simulink library "DsmCheatRead"  (R2022b)
settings: Solver=VariableStepAuto  StartTime=0.0  StopTime=10.0  RelTol=1e-3
values from neighbouring files (symbols this model uses):
  dsmIdentifier = dsmName    [DsmCheatReadConfig.m]
libraries: HandyTextFile x1
settings Model: Creator=kl13806  LastModifiedBy=kl13806
settings SolverCC: AlgebraicLoopSolver=TrustRegion
settings DebuggingCC: UnconnectedInputMsg=warning  UnconnectedOutputMsg=warning  UnconnectedLineMsg=warning  SFMachineParentedDataDiag=warning
settings ModelReferenceCC: EnableRefExpFcnMdlSchedulingChecks=on

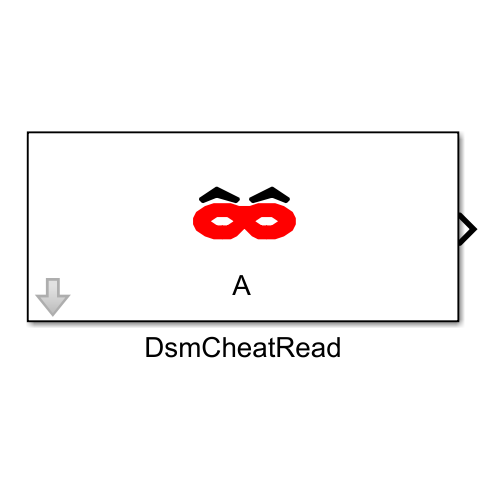
[thumbnail: Simulink's stored preview of the top-level diagram]
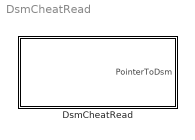
== system DsmCheatRead ==
  DsmCheatRead : Subsystem  mask{DataStoreName=A, Config=[], TriggerInit=0}
      mask prompts: DataStoreName "Simulink:blkprm_prompts:DstoreMemDstoreName"; Config "DsmCheatReadConfig"; TriggerInit "Used to trigger initialization"
      mask init:
      | blkh=gcbh;
      | Config=BTConfig.Assert(blkh,Config);
      | 
      | Config.Validate();
      | 
      | Config.DoMaskInit(blkh);
      settings: MoveFcn=DsmCheatReadConfig.CbTriggerInit(gcbh);
      mask TypeOptions DataStoreName:
      | DsmAccess/Data Store
      | Read/DataStoreName
      mask DialogControl DataStoreName Prompt: Data store name:
      mask DialogControl InfoText Prompt: Registered DSM:
      mask DialogControl RegisteredDsmName Prompt: A
      mask DialogControl ButtonRegister Prompt: Re-register DSM
      mask DialogControl ButtonRegister Callback: DsmCheatReadConfig.CbButtonRegister(gcbh);
      mask Display:
      | % retrieve icon definition
      | [path,w,h] = DsmCheatReadConfig.Icon();
      | 
      | % retrieve the block's pixel size
      | pos = get(gcbh,'position');
      | bw = pos(3) - pos(1);
      | bh = pos(4) - pos(2);
      | 
      | % draw centered icon
      | xAdj = bw/2 - w/2;
      | yAdj = bh/2 - h/2 + 5;
      | for i=1:length(path)
      |    if (path(i).rgb(1) >= 0)
      |       patch(path(i).x+xAdj, path(i).y+yAdj, path(i).rgb);
      |    end
      |    if (path(i).stroke(1) >= 0)
      |       plot(path(i).x+xAdj, path(i).y+yAdj);
      |    end
      | end
      | 
      | % show the name or an X
      | if (true)
      |     text(bw*0.5, bh*0.2, DataStoreName, 'horizontalAlignment','center');
      | 	patch(0,0,[1 1 1]);
      | 	patch(bw,bh,[1 1 1]);
      | else
      | 	tx=bw*0.03;
      | 	ty=bh*0.03;
      | 	patch([0 tx bw bw-tx], [ty 0 bh-ty bh], [1 0 0]);
      | 	patch([0 bw-tx bw tx], [bh-ty 0 ty bh], [1 0 0]);
      | end

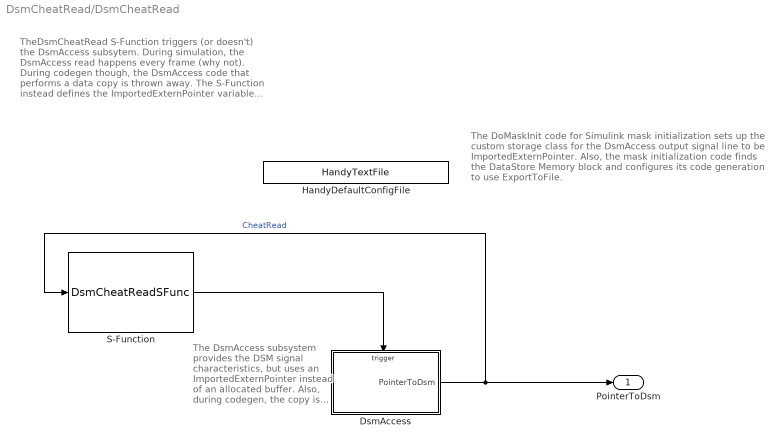
== system DsmCheatRead/DsmCheatRead ==
  note: The DsmAccess subsystem
      | provides the DSM signal
      | characteristics, but uses an
      | ImportedExternPointer instead
      | of an allocated buffer. Also,
      | during codegen, the copy is
      | never rendered to code.
  note: TheDsmCheatRead S-Function triggers (or doesn't) the DsmAccess subsytem. During simulation, the DsmAccess read happens every frame (why not). During codegen though, the DsmAccess code that performs a data copy is thrown away. The S-Function instead defines the ImportedExternPointer variable referenced at the output of the DsmAccess and assigns it to point directly to the DataStore Memory itself. The trick requires the DsmAccess output signal as an input to the SFunc just to discover its datatype and variable name. Also generated code hazards a guess at the DSM variable name in collaboration with Mask Init code that sets up the DSM to be a simple ExportToFile storage class.
  note: The DoMaskInit code for Simulink mask initialization
      | sets up the custom storage class for the DsmAccess
      | output signal line to be ImportedExternPointer. Also,
      | the mask initialization code finds the DataStore Memory
      | block and configures its code generation to use ExportToFile.
  DsmAccess : Subsystem
  HandyDefaultConfigFile : HandyTextFile/HandyTextFile  TemplateSource=Config  FileSuffix=Init  OpenDialogOnLoad=off  UseThisBlockName=off  AddGrandParentNamePrefix=off  TheDefaultText=|  ShowInLibBrowser=on
      | % $(FILENAME) Setup model parameters for each "Init" callback (e.g. update diagram)
      | sample_rate_in_hertz = 44100;
      | frame_size = 32;
      | sysin_channel_count = 2;
      settings: SourceProductName=Bose Talaria
  S-Function : S-Function  FunctionName=DsmCheatReadSFunc  Parameters=dsmIdentifier,0  SFunctionDeploymentMode=off  EnableBusSupport=off
  PointerToDsm : Outport
  wires:
  S-Function/1 -> DsmAccess/Trigger
  DsmAccess/1(PointerToDsm) -> S-Function/1, PointerToDsm/1  "CheatRead"

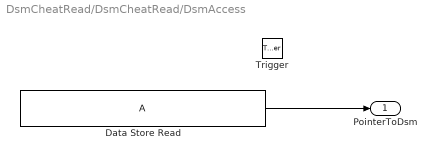
== system DsmCheatRead/DsmCheatRead/DsmAccess ==
  Trigger : TriggerPort  TriggerType=function-call  VariantControl=Variant  PortDimensions=1
  Data Store Read : DataStoreRead  IndexOptions=Index vector (dialog)  Indices=1  OutputSizes=1
  PointerToDsm : Outport
  wires:
  Data Store Read/1 -> PointerToDsm/1
